simulink model "p4_2_0"  (R2016a)
settings: Solver=VariableStepAuto  StartTime=0.0  StopTime=100.0  RelTol=1e-3
settings Model: Creator=maximilian  LastModifiedBy=maximilian

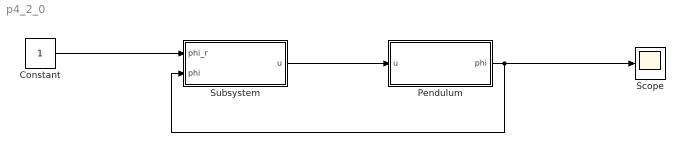
== system p4_2_0 ==
  Constant : Constant
  Pendulum : Subsystem
  Scope : Scope
  Subsystem : Subsystem
  wires:
  Subsystem/1(u) -> Pendulum/1("u ")
  Pendulum/1(phi) -> Scope/1, Subsystem/2(phi)
  Constant/1 -> Subsystem/1(phi_r)

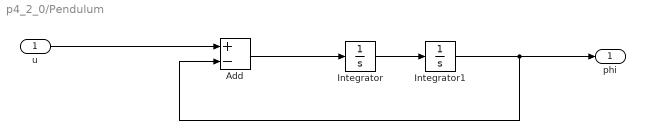
== system p4_2_0/Pendulum ==
  "u " : Inport
  Add : Sum  Inputs=+-
  Integrator : Integrator
  Integrator1 : Integrator
  phi : Outport
  wires:
  "u "/1 -> Add/1
  Add/1 -> Integrator/1
  Integrator/1 -> Integrator1/1
  Integrator1/1 -> Add/2, phi/1

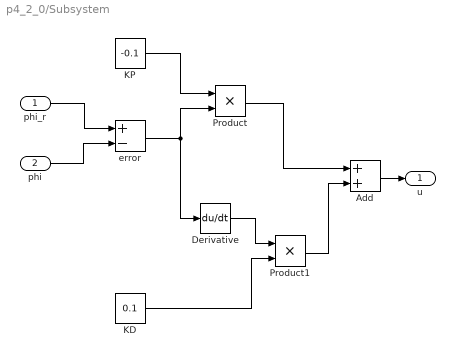
== system p4_2_0/Subsystem ==
  phi_r : Inport
  phi : Inport  Port=2
  Add : Sum
  Derivative : Derivative
  KD : Constant  Value=0.1
  KP : Constant  Value=-0.1
  Product : Product
  Product1 : Product
  error : Sum  Inputs=+-
  u : Outport
  wires:
  phi_r/1 -> error/1
  phi/1 -> error/2
  error/1 -> Derivative/1, Product/2
  KP/1 -> Product/1
  Product/1 -> Add/1
  Add/1 -> u/1
  KD/1 -> Product1/2
  Derivative/1 -> Product1/1
  Product1/1 -> Add/2
